simulink model "ex_mass_spring_simulink"  (R2024a)
settings: Solver=VariableStepAuto  StartTime=0.0  StopTime=15  RelTol=1e-3

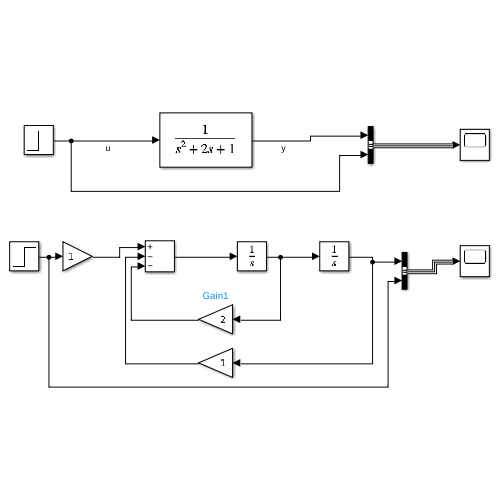
[thumbnail: Simulink's stored preview of the top-level diagram]
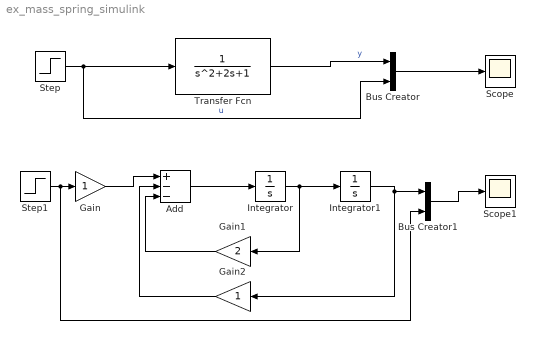
== system ex_mass_spring_simulink ==
  Add : Sum  Inputs=+--
  Bus Creator : BusCreator  Inputs=2
  Bus Creator1 : BusCreator  Inputs=2
  Gain : Gain
  Gain1 : Gain  Gain=2
  Gain2 : Gain
  Integrator : Integrator
  Integrator1 : Integrator
  Scope : Scope
  Scope1 : Scope
  Step : Step  SampleTime=0
  Step1 : Step  SampleTime=0
  Transfer Fcn : TransferFcn
  wires:
  Bus Creator/1 -> Scope/1
  Step/1 -> Bus Creator/2, Transfer Fcn/1  "u"
  Transfer Fcn/1 -> Bus Creator/1  "y"
  Integrator/1 -> Gain1/1, Integrator1/1
  Step1/1 -> Bus Creator1/2, Gain/1
  Gain/1 -> Add/1
  Gain1/1 -> Add/3
  Integrator1/1 -> Bus Creator1/1, Gain2/1
  Gain2/1 -> Add/2
  Add/1 -> Integrator/1
  Bus Creator1/1 -> Scope1/1
